simulink model "UrbanPHIL"  (Simulink 8.1)
settings: Solver=ode1  StartTime=0.0  StopTime=inf  FixedStep=Ts  MaxStep=1e-3  RelTol=1e-3
PostLoadFcn:
  | NREL_Mode=1; BANSHEE_init;
InitFcn:
  | NREL_Mode=1; BANSHEE_init;
values from neighbouring files (symbols this model uses):
  Ts = 100E-6    (= 0.0001)    [BANSHEE_init.m]    (also in Ghost_init.m)
undefined symbols (not defined in the file or in its folder): Hydride, Left, Metal, Nickel, type, V
libraries: powerlib x50, rteventslib x26, rtio_opalrt_op5142ex1 x25, artemis x13, simulink x6, cables_lib x4, relay_housing_lib x3, rtlab x2, utility_service_lib x1, Feeder1_lib x1, Feeder2_lib x1, Feeder3_lib x1
(part 1 of 3)
settings Model: ARTEMISmethode_block_infos=$$__separator__$$UrbanPHIL/ARTEMIS Guide$$__separator__$$  Creator=RE25624  LastModifiedBy=pkoralew  BufferReuse=off
settings SolverCC: ZeroCrossAlgorithm=Adaptive
settings DataIOCC: ExternalInput=getinputstruct(op_snapshot1)  InitialState=getstatestruct(op_snapshot1)  LimitDataPoints=off  MaxDataPoints=90060  SignalLoggingSaveFormat=Dataset  SaveOutput=off  SignalLogging=off  DSMLogging=off  SaveTime=off  OutputSaveName=result
settings OptimizationCC: BlockReduction=off  OptimizeBlockIOStorage=off  BufferReuse=off  ExpressionFolding=off  LocalBlockOutputs=off
settings DebuggingCC: MaxConsecutiveZCsMsg=warning  IgnoredZcDiagnostic=none  SolverPrmCheckMsg=none  MultiTaskRateTransMsg=warning  FcnCallInpInsideContextMsg=EnableAllAsWarning  FrameProcessingCompatibilityMsg=error  ModelReferenceExtraNoncontSigs=warning  StrictBusMsg=None
settings ModelReferenceCC: UpdateModelReferenceTargets=IfOutOfDate
settings SFSimCC: SFSimEcho=off
settings GRTTargetCC: CodeReplacementLibrary=C89/C90 (ANSI)

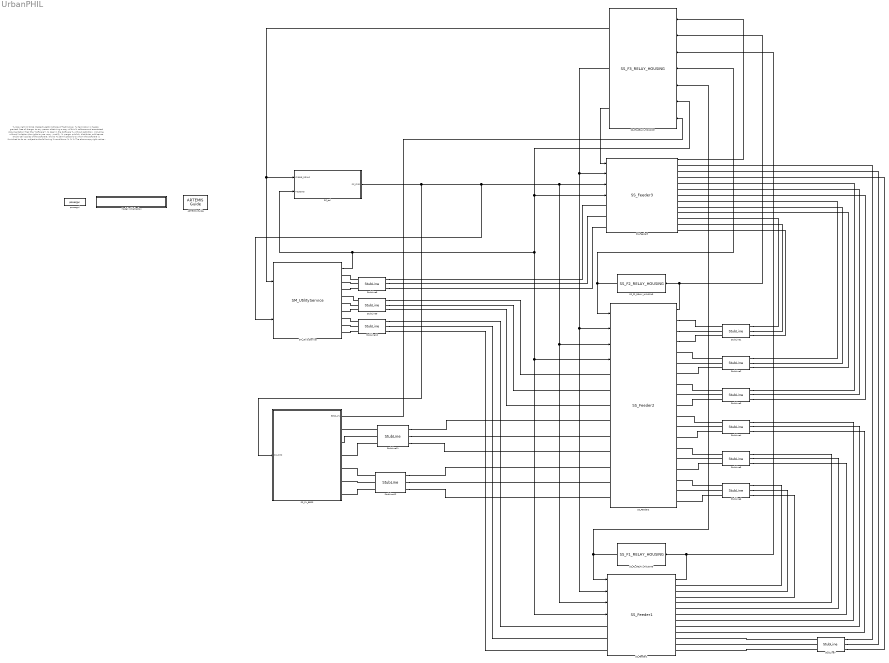
== system UrbanPHIL ==
  note: % Copyright (c) 2016 Massachusetts Institute of Technology
      | % Permission is hereby granted, free of charge, to any person obtaining a copy of this
      | % software and associated documentation files (the "Software"), to deal in the Software
      | % without restriction, including without limitation the rights to use, copy, modify,
      | % merge, publish, distribute, sublicense, and/or sell copies of the Software, and to
      | % permit persons to whom the Software is furnished to do so, subject to the following
      | % conditions:
      | %
      | %
      | % The above copyright notice and this permission notice shall be included in
      | % all copies or substantial portions of the Software.
      | %
      | % THE SOFTWARE IS PROVIDED "AS IS", WITHOUT WARRANTY OF ANY KIND, EXPRESS OR IMPLIED,
      | % INCLUDING BUT NOT LIMITED TO THE WARRANTIES OF MERCHANTABILITY, FITNESS FOR A
      | % PARTICULAR PURPOSE AND NONINFRINGEMENT. IN NO EVENT SHALL THE AUTHORS OR COPYRIGHT
      | % HOLDERS BE LIABLE FOR ANY CLAIM, DAMAGES OR OTHER LIABILITY, WHETHER IN AN ACTION
      | % OF CONTRACT, TORT OR OTHERWISE, ARISING FROM, OUT OF OR IN CONNECTION WITH THE
      | % SOFTWARE OR THE USE OR OTHER DEALINGS IN THE SOFTWARE.
      | %
      | %
      | %%
  ARTEMIS Guide : artemis/ARTEMIS/ARTEMIS Guide  Tag=FTSSmethode_opal_4hx0r99  Description=5.0_z1  lock=on  Ts=Ts  opt=art5  dyna=off  nb_perm=4  RT_fullcomp=off  ssn=on  ssn_itvc=off  ssn_ivic=off  ssn_ext=off  ssn_solver=Art5 with Backward Euler nodal interface  ssn_impulse=off  ssn_quasimpulse=off  ssn_impulse_loop=5  paraExtinctionThy=off  Thy_Impulse=on  dtc=Off  dtc_opt=normal  ao=on  simtype=off  ct_mac=off  lin_mov=off  lsp=[0.001 2]  spike_skip=Disabled  dtc_extra=1  dtc_sws=normal  dtc_pied=0.5  SPSRulesBlock=SPSRules  tre=on  ctmm=off  LF=off  dpl_type=ARTEMiS DPL  rlc_type=off  custom_type=off  para=on  ssn_ImpulseLoopBlockedStateUpdate=5  ssn_mov_iter_number=5  ssn_switch_iter_number=5
  Model Initialization : Subsystem  AncestorBlock=artemis/Tools /Misc/Model Initialization  mask(Model Functions){InitFcnX=NREL_Mode=1; BANSHEE_init;, prel=off, posl=on, inif=on, strf=off}
      mask prompts: InitFcnX "Initialisation"; prel "Preload Function"; posl "PostLoad Function"; inif "InitFcn"; strf "StartFcn"
      mask init:
      | currentBlock = gcb;
      | root = bdroot(currentBlock);
      | 
      | if ~strcmp(get_param(root,'BlockDiagramType'),'library')
      |     if prel==1
      |         set_param(root, 'PreLoadFcn', InitFcnX);
      |     else
      |         set_param(root, 'PreLoadFcn', '');
      |     end
      |     if inif==1
      |         set_param(root, 'InitFcn', InitFcnX);
      |     else
      |         set_param(root, 'InitFcn', '');
      |     end
      |     if strf==1
      |         set_param(root, 'StartFcn', InitFcnX);
      |     else
      |         set_param(root, 'StartFcn', '');
      |     end
      |     if posl==1
      |         set_param(root, 'PostLoadFcn', InitFcnX);
      |     else
      |         set_param(root, 'PostLoadFcn', '');
      |     end
      | end
      | 
      | pos = get_param(currentBlock, 'Position');
      | width = pos(3) - pos(1); height = pos(4) - pos(2);
      | txt = [ upper(root) '\n' '- InitFcn. . . . . '  get_param(root, 'InitFcn') ];
      settings: CopyFcn=set_param(gcb,'LinkStatus','inactive')
      mask Display: text(5, height*0.5, txt, 'horizontalAlignment', 'left', 'verticalAlignment', 'middle') ;
  SC_ctrl : Subsystem
  SM_UtilityService : utility_service_lib/SM_UtilityService
  SS_F1_RELAY_HOUSING : relay_housing_lib/SS_F1_RELAY_HOUSING
  SS_F2_RELAY_HOUSING : relay_housing_lib/SS_F2_RELAY_HOUSING
  SS_F3_RELAY_HOUSING : relay_housing_lib/SS_F3_RELAY_HOUSING
  SS_Feeder1 : Feeder1_lib/SS_Feeder1
  SS_Feeder2 : Feeder2_lib/SS_Feeder2
  SS_Feeder3 : Feeder3_lib/SS_Feeder3
  SS_PV_BESS : Subsystem
  StubLine1 : artemis/ARTEMIS/StubLine  Phases=3  pu=off  L=1500 * 9.43453e-08 / 2  Lpu=0.08  R=1500 * 2.28409e-5 / 2  Rpu=0.002  S_base=450e6/3  V_base=230e3/sqrt(3)  F_base=60  Ts=Ts
  StubLine10 : artemis/ARTEMIS/StubLine  Phases=3  pu=on  L=1500 * 9.43453e-08 / 2  Lpu=0.08  R=1500 * 2.28409e-5 / 2  Rpu=0.002  S_base=50e6/3  V_base=13.8e3/sqrt(3)  F_base=60  Ts=Ts
  StubLine11 : artemis/ARTEMIS/StubLine  Phases=3  pu=off  L=100 * 9.43453e-08  Lpu=0.08  R=100 * 2.28409e-5  Rpu=0.002  S_base=450e6/3  V_base=230e3/sqrt(3)  F_base=60  Ts=Ts
  StubLine12 : artemis/ARTEMIS/StubLine  Phases=3  pu=off  L=100 * 9.43453e-08  Lpu=0.08  R=100 * 2.28409e-5  Rpu=0.002  S_base=450e6/3  V_base=230e3/sqrt(3)  F_base=60  Ts=Ts
  StubLine2 : artemis/ARTEMIS/StubLine  Phases=3  pu=off  L=1500 * 9.43453e-08 / 2  Lpu=0.08  R=1500 * 2.28409e-5 / 2  Rpu=0.002  S_base=450e6/3  V_base=230e3/sqrt(3)  F_base=60  Ts=Ts
  StubLine3 : artemis/ARTEMIS/StubLine  Phases=3  pu=off  L=1500 * 9.43453e-08 / 2  Lpu=0.08  R=1500 * 2.28409e-5 / 2  Rpu=0.002  S_base=450e6/3  V_base=230e3/sqrt(3)  F_base=60  Ts=Ts
  StubLine4 : artemis/ARTEMIS/StubLine  Phases=3  pu=off  L=1000 * 9.43453e-08 / 2  Lpu=0.08  R=1000 * 2.28409e-5 / 2  Rpu=0.002  S_base=450e6/3  V_base=230e3/sqrt(3)  F_base=60  Ts=Ts
  StubLine5 : artemis/ARTEMIS/StubLine  Phases=3  pu=off  L=2000 * 9.43453e-08 / 2  Lpu=0.08  R=2000 * 2.28409e-5 / 2  Rpu=0.002  S_base=450e6/3  V_base=230e3/sqrt(3)  F_base=60  Ts=Ts
  StubLine6 : artemis/ARTEMIS/StubLine  Phases=3  pu=off  L=2000 * 9.43453e-08 / 2  Lpu=0.08  R=2000 * 2.28409e-5 / 2  Rpu=0.002  S_base=450e6/3  V_base=230e3/sqrt(3)  F_base=60  Ts=Ts
  StubLine7 : artemis/ARTEMIS/StubLine  Phases=3  pu=off  L=2000 * 9.43453e-08 / 2  Lpu=0.08  R=2000 * 2.28409e-5 / 2  Rpu=0.002  S_base=450e6/3  V_base=230e3/sqrt(3)  F_base=60  Ts=Ts
  StubLine8 : artemis/ARTEMIS/StubLine  Phases=3  pu=on  L=1500 * 9.43453e-08 / 2  Lpu=0.08  R=1500 * 2.28409e-5 / 2  Rpu=0.002  S_base=50e6/3  V_base=13.8e3/sqrt(3)  F_base=60  Ts=Ts
  StubLine9 : artemis/ARTEMIS/StubLine  Phases=3  pu=on  L=1500 * 9.43453e-08 / 2  Lpu=0.08  R=1500 * 2.28409e-5 / 2  Rpu=0.002  S_base=50e6/3  V_base=13.8e3/sqrt(3)  F_base=60  Ts=Ts
  powergui : powerlib/powergui  Priority=2  SimulationMode=Discrete  SolverType=Tustin  SampleTime=Ts  frequency=60  SPID=off  DisableSnubberDevices=off  DisableRonSwitches=off  DisableVfSwitches=off  SwTol=0  Interpol=off  DisplayEquations=off  frequencyindice=0  Pbase=100e6  ErrMax=1e-4  Iterations=50  UnitsV=kV  UnitsW=MW  FunctionMessages=off  echomessages=off  HookPort=off  EnableUseOfTLC=off  x0status=blocks  RestoreLinks=warning  ResistiveCurrentMeasurement=off  Frange=logspace(0,3,50)  Ylog=off  Xlog=off  ShowGrid=off  save=off  variable=ZData  structure=0  ZoomFFT=on  StartTime=0.0  cycles=2  DisplayStyle=off  fundamental=60  FreqAxis=off  MaxFrequency=1000  frequencyindicesteady=1  RmsSteady=1  display=off  Ts=0  methode=off
  wires:
  SS_Feeder3/1 -> SS_F3_RELAY_HOUSING/1
  SS_F3_RELAY_HOUSING/3 -> SS_Feeder3/1
  SS_F1_RELAY_HOUSING/1 -> SS_F3_RELAY_HOUSING/5, SS_Feeder1/1
  SS_F2_RELAY_HOUSING/1 -> SS_F3_RELAY_HOUSING/4, SS_Feeder2/1
  SS_Feeder1/1 -> SS_F3_RELAY_HOUSING/3, SS_F1_RELAY_HOUSING/1
  SS_Feeder2/1 -> SS_F3_RELAY_HOUSING/2, SS_F2_RELAY_HOUSING/1
  SS_F3_RELAY_HOUSING/2 -> SS_Feeder1/2, SS_Feeder2/2, SS_Feeder3/2
  SM_UtilityService/1 -> SC_ctrl/2(TestData), SS_Feeder1/4, SS_Feeder2/4, SS_F3_RELAY_HOUSING/6, SS_Feeder3/4
  SS_F3_RELAY_HOUSING/1 -> SC_ctrl/1(CMBNE_SGNLS), SM_UtilityService/1
  SC_ctrl/1(SC_CMD) -> SS_PV_BESS/1(SC_CMD), SM_UtilityService/2, SS_Feeder1/3, SS_Feeder2/3, SS_Feeder3/3
  SS_PV_BESS/1(BESS_PV) -> SS_F3_RELAY_HOUSING/7
  connections:
  SS_Feeder2/RConn2 -- StubLine1/LConn2
  SS_Feeder2/RConn1 -- StubLine1/LConn1
  SS_Feeder2/RConn3 -- StubLine1/LConn3
  StubLine2/LConn2 -- SS_Feeder2/RConn5
  StubLine2/LConn3 -- SS_Feeder2/RConn6
  StubLine2/LConn1 -- SS_Feeder2/RConn4
  StubLine3/LConn2 -- SS_Feeder2/RConn8
  StubLine3/LConn1 -- SS_Feeder2/RConn7
  StubLine3/LConn3 -- SS_Feeder2/RConn9
  StubLine4/LConn3 -- SS_Feeder2/RConn12
  StubLine4/LConn2 -- SS_Feeder2/RConn11
  StubLine4/LConn1 -- SS_Feeder2/RConn10
  StubLine7/LConn3 -- SS_Feeder1/RConn12
  StubLine7/LConn2 -- SS_Feeder1/RConn11
  StubLine7/LConn1 -- SS_Feeder1/RConn10
  StubLine5/LConn2 -- SS_Feeder2/RConn14
  StubLine5/LConn1 -- SS_Feeder2/RConn13
  StubLine5/LConn3 -- SS_Feeder2/RConn15
  StubLine6/LConn3 -- SS_Feeder2/RConn18
  StubLine6/LConn2 -- SS_Feeder2/RConn17
  StubLine6/LConn1 -- SS_Feeder2/RConn16
  StubLine6/RConn1 -- SS_Feeder1/RConn1
  StubLine6/RConn2 -- SS_Feeder1/RConn2
  StubLine6/RConn3 -- SS_Feeder1/RConn3
  StubLine5/RConn1 -- SS_Feeder1/RConn4
  StubLine5/RConn2 -- SS_Feeder1/RConn5
  StubLine5/RConn3 -- SS_Feeder1/RConn6
  StubLine4/RConn1 -- SS_Feeder1/RConn7
  StubLine4/RConn2 -- SS_Feeder1/RConn8
  StubLine4/RConn3 -- SS_Feeder1/RConn9
  StubLine3/RConn3 -- SS_Feeder3/RConn6
  StubLine3/RConn2 -- SS_Feeder3/RConn5
  StubLine3/RConn1 -- SS_Feeder3/RConn4
  StubLine2/RConn3 -- SS_Feeder3/RConn9
  StubLine2/RConn2 -- SS_Feeder3/RConn8
  StubLine2/RConn1 -- SS_Feeder3/RConn7
  StubLine1/RConn3 -- SS_Feeder3/RConn12
  StubLine1/RConn2 -- SS_Feeder3/RConn11
  StubLine1/RConn1 -- SS_Feeder3/RConn10
  StubLine7/RConn1 -- SS_Feeder3/RConn1
  StubLine7/RConn2 -- SS_Feeder3/RConn2
  StubLine7/RConn3 -- SS_Feeder3/RConn3
  StubLine8/LConn1 -- SM_UtilityService/RConn1
  StubLine8/LConn2 -- SM_UtilityService/RConn2
  StubLine8/LConn3 -- SM_UtilityService/RConn3
  StubLine9/LConn2 -- SM_UtilityService/RConn5
  StubLine9/LConn3 -- SM_UtilityService/RConn6
  StubLine9/LConn1 -- SM_UtilityService/RConn4
  StubLine10/LConn2 -- SM_UtilityService/RConn8
  StubLine10/LConn3 -- SM_UtilityService/RConn9
  StubLine10/LConn1 -- SM_UtilityService/RConn7
  StubLine8/RConn3 -- SS_Feeder3/LConn3
  StubLine8/RConn2 -- SS_Feeder3/LConn2
  StubLine8/RConn1 -- SS_Feeder3/LConn1
  StubLine10/RConn1 -- SS_Feeder1/LConn1
  StubLine10/RConn2 -- SS_Feeder1/LConn2
  StubLine10/RConn3 -- SS_Feeder1/LConn3
  StubLine9/RConn1 -- SS_Feeder2/LConn1
  StubLine9/RConn2 -- SS_Feeder2/LConn2
  StubLine9/RConn3 -- SS_Feeder2/LConn3
  StubLine11/LConn2 -- SS_PV_BESS/RConn2
  StubLine11/LConn1 -- SS_PV_BESS/RConn1
  StubLine11/LConn3 -- SS_PV_BESS/RConn3
  StubLine11/RConn2 -- SS_Feeder2/LConn5
  StubLine11/RConn3 -- SS_Feeder2/LConn6
  StubLine11/RConn1 -- SS_Feeder2/LConn4
  StubLine12/LConn2 -- SS_PV_BESS/RConn5
  StubLine12/LConn1 -- SS_PV_BESS/RConn4
  StubLine12/LConn3 -- SS_PV_BESS/RConn6
  StubLine12/RConn2 -- SS_Feeder2/LConn8
  StubLine12/RConn1 -- SS_Feeder2/LConn7
  StubLine12/RConn3 -- SS_Feeder2/LConn9

== system UrbanPHIL/Model Initialization ==

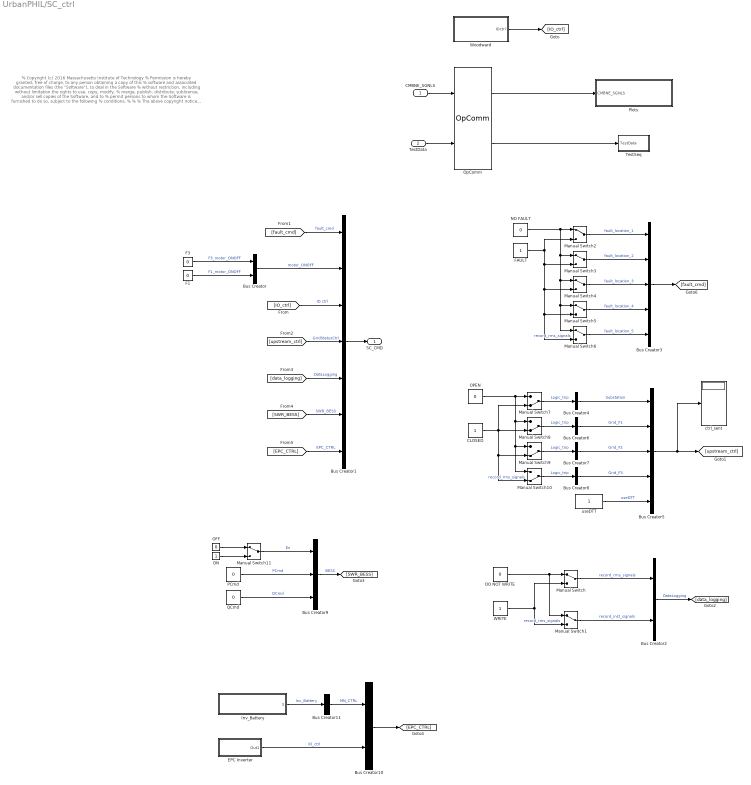
== system UrbanPHIL/SC_ctrl ==
  note: % Copyright (c) 2016 Massachusetts Institute of Technology
      | % Permission is hereby granted, free of charge, to any person obtaining a copy of this
      | % software and associated documentation files (the "Software"), to deal in the Software
      | % without restriction, including without limitation the rights to use, copy, modify,
      | % merge, publish, distribute, sublicense, and/or sell copies of the Software, and to
      | % permit persons to whom the Software is furnished to do so, subject to the following
      | % conditions:
      | %
      | %
      | % The above copyright notice and this permission notice shall be included in
      | % all copies or substantial portions of the Software.
      | %
      | % THE SOFTWARE IS PROVIDED "AS IS", WITHOUT WARRANTY OF ANY KIND, EXPRESS OR IMPLIED,
      | % INCLUDING BUT NOT LIMITED TO THE WARRANTIES OF MERCHANTABILITY, FITNESS FOR A
      | % PARTICULAR PURPOSE AND NONINFRINGEMENT. IN NO EVENT SHALL THE AUTHORS OR COPYRIGHT
      | % HOLDERS BE LIABLE FOR ANY CLAIM, DAMAGES OR OTHER LIABILITY, WHETHER IN AN ACTION
      | % OF CONTRACT, TORT OR OTHERWISE, ARISING FROM, OUT OF OR IN CONNECTION WITH THE
      | % SOFTWARE OR THE USE OR OTHER DEALINGS IN THE SOFTWARE.
      | %
      | %
      | %%
  CMBNE_SGNLS : Inport
  TestData : Inport  Port=2
  Bus Creator : BusCreator  Inputs=2
  Bus Creator1 : BusCreator  Inputs=7
  Bus Creator10 : BusCreator  Inputs=2
  Bus Creator{4,6..8,11} (5 alike) : BusCreator  Inputs=1
  Bus Creator2 : BusCreator  Inputs=2
  Bus Creator3 : BusCreator  Inputs=5
  Bus Creator5 : BusCreator  Inputs=5
  Bus Creator9 : BusCreator  Inputs=3
  CLOSED : Constant
  DO NOT WRITE : Constant  Value=0
  EPC Inverter : Subsystem
  F1 : Constant  Value=0
  F3 : Constant  Value=0
  FAULT : Constant
  Inv_Battery : Subsystem
  Manual Switch{,1..6,11} (8 alike) : ManualSwitch
  Manual Switch{7..10} (4 alike) : ManualSwitch  CurrentSetting=0
  NO FAULT : Constant  Value=0
  OFF : Constant  Value=0
  ON : Constant
  OPEN : Constant  Value=0
  OpComm : rtlab/OpComm  nbport=2  groupe_acq=1  subsys_rate=0  st=0  Synchronization=on  Interpolation=on  Threshold=1.0  Missed_Data=off  Sim_Time=off  Samples=off  dynSigOut=off  from_console=0  warning_done=off  writeOpCommFile=off  Offset=off
  PCmd : Constant  Value=0  SampleTime=Ts
  Plots : Subsystem
  QCmd : Constant  Value=0  SampleTime=Ts
  TestSeq : Subsystem
  WRITE : Constant
  Woodward : Subsystem
  ctrl_sent : Display
  useDTT : Constant
  SC_CMD : Outport
  wires:
  CMBNE_SGNLS/1 -> OpComm/1
  Bus Creator1/1 -> SC_CMD/1
  [IO_ctrl] -> Bus Creator1/3  "IO ctrl"
  Woodward/1(IOctrl) -> [IO_ctrl]
  [fault_cmd] -> Bus Creator1/1  "fault_cmd"
  Bus Creator/1 -> Bus Creator1/2  "motor_ONOFF"
  F3/1 -> Bus Creator/1  "F3_motor_ONOFF"
  F1/1 -> Bus Creator/2  "F1_motor_ONOFF"
  [upstream_ctrl] -> Bus Creator1/4  "GridStatusCtrl"
  Manual Switch/1 -> Bus Creator2/1  "record_rms_signals"
  Manual Switch1/1 -> Bus Creator2/2  "record_inst_signals"
  Bus Creator2/1 -> [data_logging]  "DataLogging"
  OpComm/1 -> Plots/1(CMBNE_SGNLS)
  OpComm/2 -> TestSeq/1(TestData)
  TestData/1 -> OpComm/2
  WRITE/1 -> Manual Switch1/2, Manual Switch/2  "record_rms_signals"
  DO NOT WRITE/1 -> Manual Switch1/1, Manual Switch/1
  Bus Creator3/1 -> [fault_cmd]
  Manual Switch2/1 -> Bus Creator3/1  "fault_location_1"
  Manual Switch6/1 -> Bus Creator3/5  "fault_location_5"
  Manual Switch3/1 -> Bus Creator3/2  "fault_location_2"
  Manual Switch4/1 -> Bus Creator3/3  "fault_location_3"
  Manual Switch5/1 -> Bus Creator3/4  "fault_location_4"
  NO FAULT/1 -> Manual Switch6/1, Manual Switch5/1, Manual Switch4/1, Manual Switch3/1, Manual Switch2/1
  FAULT/1 -> Manual Switch2/2, Manual Switch6/2, Manual Switch5/2, Manual Switch4/2, Manual Switch3/2  "record_rms_signals"
  Manual Switch10/1 -> Bus Creator8/1  "Logic_trip"
  Manual Switch9/1 -> Bus Creator7/1  "Logic_trip"
  Bus Creator5/1 -> ctrl_sent/1, [upstream_ctrl]
  Manual Switch8/1 -> Bus Creator6/1  "Logic_trip"
  Bus Creator4/1 -> Bus Creator5/1  "Substation"
  Manual Switch7/1 -> Bus Creator4/1  "Logic_trip"
  Bus Creator8/1 -> Bus Creator5/4  "Grid_F3"
  Bus Creator7/1 -> Bus Creator5/3  "Grid_F2"
  Bus Creator6/1 -> Bus Creator5/2  "Grid_F1"
  useDTT/1 -> Bus Creator5/5  "useDTT"
  OPEN/1 -> Manual Switch7/1, Manual Switch8/1, Manual Switch9/1, Manual Switch10/1
  CLOSED/1 -> Manual Switch7/2, Manual Switch8/2, Manual Switch9/2, Manual Switch10/2  "record_rms_signals"
  Manual Switch11/1 -> Bus Creator9/1  "En"
  PCmd/1 -> Bus Creator9/2  "PCmd"
  QCmd/1 -> Bus Creator9/3  "QCmd"
  ON/1 -> Manual Switch11/2
  OFF/1 -> Manual Switch11/1
  [data_logging] -> Bus Creator1/5  "DataLogging"
  Bus Creator9/1 -> [SWR_BESS]  "BESS"
  [SWR_BESS] -> Bus Creator1/6  "SWR_BESS"
  EPC Inverter/1(Out1) -> Bus Creator10/2  "IO_ctrl"
  Inv_Battery/1(S) -> Bus Creator11/1  "Inv_Battery"
  Bus Creator11/1 -> Bus Creator10/1  "MN_CTRL"
  Bus Creator10/1 -> [EPC_CTRL]
  [EPC_CTRL] -> Bus Creator1/7  "EPC_CTRL"

== system UrbanPHIL/SS_PV_BESS ==
  SC_CMD : Inport
  BESS : BESS_lib/BESS
  Bus Creator6 : BusCreator  Inputs=2
  Bus Selector7 : BusSelector  OutputSignals=SWR_BESS,EPC_CTRL
  C1 : cables_lib/500kcmil-Mutual  length=10  par_sets=1  ratio=3
  C202 : cables_lib/500kcmil-Mutual  length=10  par_sets=1  ratio=3
  EPC : Subsystem
  Memory : Memory
  OpComm3 : rtlab/OpComm  nbport=1  groupe_acq=1  subsys_rate=0  st=0  Synchronization=on  Interpolation=on  Threshold=1.0  Missed_Data=off  Sim_Time=off  Samples=off  dynSigOut=off  from_console=1  warning_done=off  writeOpCommFile=off  Offset=off
  A_PV : PMIOPort  Port=1  Side=Right
  B_PV : PMIOPort  Port=2  Side=Right
  C_PV : PMIOPort  Port=3  Side=Right
  A_BESS : PMIOPort  Port=4  Side=Right
  B_BESS : PMIOPort  Port=5  Side=Right
  C_BESS : PMIOPort  Port=6  Side=Right
  BESS_PV : Outport
  wires:
  SC_CMD/1 -> OpComm3/1
  OpComm3/1 -> Bus Selector7/1
  Bus Selector7/1 -> [SWR_BESS]  "<SWR_BESS>"
  [SWR_BESS] -> BESS/1
  BESS/1 -> [BESS_MS]
  Memory/1 -> BESS_PV/1
  Bus Creator6/1 -> Memory/1
  [BESS_MS] -> Bus Creator6/1  "BESS"
  EPC/1(monitoring) -> [EPC_MS]
  [EPC_MS] -> Bus Creator6/2  "EPC"
  [EPC_CTRL] -> EPC/1(FROM_SC)
  Bus Selector7/2 -> [EPC_CTRL]  "<EPC_CTRL>"
  connections:
  B_BESS/RConn1 -- C1/RConn2
  C_BESS/RConn1 -- C1/RConn3
  A_BESS/RConn1 -- C1/RConn1
  B_PV/RConn1 -- C202/RConn2
  C_PV/RConn1 -- C202/RConn3
  A_PV/RConn1 -- C202/RConn1
  BESS/RConn2 -- C202/LConn2
  BESS/RConn3 -- C202/LConn3
  BESS/RConn1 -- C202/LConn1
  EPC/LConn1 -- C1/LConn1
  EPC/LConn2 -- C1/LConn2
  EPC/LConn3 -- C1/LConn3

== system UrbanPHIL/SC_ctrl/EPC Inverter ==
  note: This corresponds to
      | the DIO Enable MCB
  note: Op_Mode:
      | 0 = Relay Functions
      | 1 = Close Breaker
      | 2 = Open Breaker
  16Din/16Dout GR3 : Subsystem
  16PWMIn/16PWMout GR3 : Subsystem
  16TSDIn/16 TSDOut GR3 : Subsystem
  Brk1 Grid : Constant  Value=2
  Brk10 Gen 1 Busbar : Constant
  Brk2 Load 1 : Constant  Value=0
  Brk3 Inv MX1 : Constant  Value=2
  Brk4 Gen 1 MCB : Constant  Value=2
  Brk5 Gen 2 LCB : Constant  Value=0
  Brk6 Gen 1 LCB : Constant  Value=0
  Brk7 Gen 2 GCB : Constant
  Brk8 Gen 1 GCB : Constant
  Brk9 Gen 2 Busbar : Constant
  Bus Creator1 : BusCreator  Inputs=3
  Bus Creator2 : BusCreator  Inputs=2
  Bus Creator3 : BusCreator  Inputs=14
  Wood MCB Enable : Constant  Value=0
  bias_ctrl : Constant
  control_mode : Constant
  gen_enable : Constant
  Out1 : Outport
  wires:
  Brk10 Gen 1 Busbar/1 -> Bus Creator3/10  "Gen1_Busbar"
  Brk9 Gen 2 Busbar/1 -> Bus Creator3/9  "Gen2_Busbar"
  Brk8 Gen 1 GCB/1 -> Bus Creator3/8  "Gen1_GCB"
  Brk7 Gen 2 GCB/1 -> Bus Creator3/7  "Gen2_GCB"
  Brk6 Gen 1 LCB/1 -> Bus Creator3/6  "Load 3"
  Brk5 Gen 2 LCB/1 -> Bus Creator3/5  "Load 2"
  Wood MCB Enable/1 -> Bus Creator3/14  "Wood_MCB_enable"
  Bus Creator2/1 -> Out1/1
  bias_ctrl/1 -> Bus Creator3/13  "Gen_bias_enable"
  gen_enable/1 -> Bus Creator3/12  "Gen2_enable"
  control_mode/1 -> Bus Creator3/11  "Wood_DIO"
  Brk4 Gen 1 MCB/1 -> Bus Creator3/4  "Gen1_MCB"
  Brk3 Inv MX1/1 -> Bus Creator3/3  "MX1"
  Brk2 Load 1/1 -> Bus Creator3/2  "Load 1"
  Brk1 Grid/1 -> Bus Creator3/1  "Grid"
  Bus Creator3/1 -> Bus Creator2/2  "test_controls"
  Bus Creator1/1 -> Bus Creator2/1  "DOUT GR3"
  16PWMIn/16PWMout GR3/1(To PWMOut) -> Bus Creator1/3  "16 PWMOUT GR3"
  16TSDIn/16 TSDOut GR3/1(TSDout) -> Bus Creator1/2  "16 TSDOUT GR3"
  16Din/16Dout GR3/1(Dout) -> Bus Creator1/1  "16 DOUT GR3"

== system UrbanPHIL/SC_ctrl/Inv_Battery ==
  note: Make this 1 to allow
      | the external signals.
  note: Remote Sense =>1
      | Use Remote Sense EPyQ
      | Sync or not => grid forming/grid following
  note: 0=> Local
      | 1=> Remote
  note: 0=> No Console
      | 1=> Console Ctrl
  note: 1 => Sig 1 is Bot then Sig 2 is Top
      | 0 => Sig 1 is Top then Sig 2 is Bot
  note: 0=> RTE
      | 1=> Simulink
  note: LSB
  note: MSB
  note: 1111: RTE TSD Signal Modulation External
      | 0111: RTE Signal Modulation Internal
      | X011: Sin Tri Modulatiion Internal
      | XX01: Digital Inputs
      | XXX0; Open Switches
  note: MCB
  note: GCB
  note: 1 => Closed
      | 2=> Open
  note: ~ 2.5 sec to get
      | to rated voltage
  note: RTE Internal
      | All 0 and one 1
  note: Internal = 0
      | External = 1
  Bus Creator : BusCreator  Inputs=8
  Bus Creator1 : BusCreator  Inputs=5
  Console : Constant  Value=0
  DC Contactor : Constant  Value=0
  Enable PWM{0..3} (4 alike) : Constant
  MX1 : Constant  Value=2
  MX2 : Constant  Value=2
  Precharge : Constant  Value=0
  Sense : Constant  Value=0
  Signal Mapping : Constant
  Simulink : Constant  Value=0
  S : Outport
  wires:
  Sense/1 -> Bus Creator/8  "LOCALvsREMOTE"
  Console/1 -> Bus Creator/7  "Console_Ctrl"
  Signal Mapping/1 -> Bus Creator1/5  "Ext_PWM_RTE_Signal"
  Simulink/1 -> Bus Creator/6  "RTEvsSPS"
  Enable PWM3/1 -> Bus Creator1/1
  Enable PWM2/1 -> Bus Creator1/2
  Enable PWM1/1 -> Bus Creator1/3
  Enable PWM0/1 -> Bus Creator1/4
  Bus Creator1/1 -> Bus Creator/1  "Enable PWM"
  MX2/1 -> Bus Creator/5  "MX2"
  MX1/1 -> Bus Creator/4  "MX1"
  DC Contactor/1 -> Bus Creator/3  "DC_Contactor"
  Precharge/1 -> Bus Creator/2  "Precharge"
  Bus Creator/1 -> S/1

== system UrbanPHIL/SC_ctrl/Plots ==
  note: VRMSLL
      | Hz
      | kW
      | kVAR
  CMBNE_SGNLS : Inport
  Bus Selector1 : BusSelector  OutputSignals=F1_MS_IN.DIESEL_DATA.DIESEL_GCB.VRMSLL,F1_MS_IN.DIESEL_DATA.DIESEL_GCB.Freq,F1_MS_IN.DIESEL_DATA.DIESEL_GCB.kw,F1_MS_IN.DIESEL_DATA.DIESEL_GCB.kvar  OutputAsBus=on
  Bus Selector2 : BusSelector  OutputSignals=F3_MS_IN.NG_CHP_DATA.NG_CHP_GCB.VRMSLL,F3_MS_IN.NG_CHP_DATA.NG_CHP_GCB.Freq,F3_MS_IN.NG_CHP_DATA.NG_CHP_GCB.kw,F3_MS_IN.NG_CHP_DATA.NG_CHP_GCB.kvar  OutputAsBus=on
  Bus Selector3 : BusSelector  OutputSignals=PCC_DATA_OUT.F3_PCC.VRMSLL,PCC_DATA_OUT.F3_PCC.Freq,PCC_DATA_OUT.F3_PCC.kw,PCC_DATA_OUT.F3_PCC.kvar  OutputAsBus=on
  Bus Selector4 : BusSelector  OutputSignals=PCC_DATA_OUT.F2_PCC.VRMSLL,PCC_DATA_OUT.F2_PCC.Freq,PCC_DATA_OUT.F2_PCC.kw,PCC_DATA_OUT.F2_PCC.kvar  OutputAsBus=on
  Bus Selector5 : BusSelector  OutputSignals=PCC_DATA_OUT.F1_PCC.VRMSLL,PCC_DATA_OUT.F1_PCC.Freq,PCC_DATA_OUT.F1_PCC.kw,PCC_DATA_OUT.F1_PCC.kvar  OutputAsBus=on
  Bus Selector6 : BusSelector  OutputSignals=BESS_PV.BESS.kw,BESS_PV.BESS.kvar,BESS_PV.BESS.Freq  OutputAsBus=on
  Bus Selector7 : BusSelector  OutputSignals=BESS_PV.EPC.BESS_MX1.VRMSLL,BESS_PV.EPC.BESS_MX1.Freq,BESS_PV.EPC.BESS_MX1.kw,BESS_PV.EPC.BESS_MX1.kvar  OutputAsBus=on
  Bus Selector8 : BusSelector  OutputSignals=BESS_PV.EPC.BESS_MX1.cb_ms.Iabc,BESS_PV.EPC.BESS_MX1.cb_ms.Vabc_line
  CHP : Display
  Diesel : Display
  EPC_BESS : Display
  EPC_BESS Scope : Scope  NumInputPorts=2
      settings: YMin=-5~-5  YMax=5~5
  F1 : Display
  F2 : Display
  F3 : Display
  SWR_BESS : Display
  wires:
  Bus Selector5/1 -> F1/1
  Bus Selector4/1 -> F2/1
  Bus Selector3/1 -> F3/1
  Bus Selector1/1 -> Diesel/1
  Bus Selector2/1 -> CHP/1
  CMBNE_SGNLS/1 -> [CMBNE_SGNLS]
  [CMBNE_SGNLS] -> Bus Selector5/1
  [CMBNE_SGNLS] -> Bus Selector4/1
  [CMBNE_SGNLS] -> Bus Selector3/1
  [CMBNE_SGNLS] -> Bus Selector2/1
  [CMBNE_SGNLS] -> Bus Selector1/1
  [CMBNE_SGNLS] -> Bus Selector6/1
  Bus Selector6/1 -> SWR_BESS/1
  [CMBNE_SGNLS] -> Bus Selector7/1
  Bus Selector7/1 -> EPC_BESS/1
  [CMBNE_SGNLS] -> Bus Selector8/1
  Bus Selector8/2 -> EPC_BESS Scope/2  "<Vabc_line>"
  Bus Selector8/1 -> EPC_BESS Scope/1  "<Iabc>"

== system UrbanPHIL/SC_ctrl/TestSeq ==
  TestData : Inport
  Bus Selector : BusSelector  OutputSignals=TestSeq.TimeStamp,TestSeq.fault_location_1,TestSeq.fault_location_2,TestSeq.fault_location_3,TestSeq.fault_location_4,TestSeq.fault_location_5,TestSeq.Cut_Grid_Power,TestSeq.Irradiance,TestSeq.motor_1,TestSeq.motor_2,TestSeq.Test3
  Display : Display
  Scope : Scope  NumInputPorts=10
      settings: YMin=-5~-5~-5~-5~-5~-5~-5~-5~-5~-5  YMax=5~5~5~5~5~5~5~5~5~5
  wires:
  TestData/1 -> Bus Selector/1
  Bus Selector/1 -> Display/1  "<TimeStamp>"
  Bus Selector/6 -> Scope/5  "<fault_location_5>"
  Bus Selector/5 -> Scope/4  "<fault_location_4>"
  Bus Selector/10 -> Scope/9  "<motor_2>"
  Bus Selector/2 -> Scope/1  "<fault_location_1>"
  Bus Selector/3 -> Scope/2  "<fault_location_2>"
  Bus Selector/8 -> Scope/7  "<Irradiance>"
  Bus Selector/9 -> Scope/8  "<motor_1>"
  Bus Selector/4 -> Scope/3  "<fault_location_3>"
  Bus Selector/7 -> Scope/6  "<Cut_Grid_Power>"
  Bus Selector/11 -> Scope/10  "<Test3>"

== system UrbanPHIL/SC_ctrl/Woodward ==
  16Din/16Dout GR3 : Subsystem
  Bus Creator2 : BusCreator  Inputs=1
  IOctrl : Outport
  wires:
  16Din/16Dout GR3/1(Dout) -> Bus Creator2/1  "16 DOUT GR3"
  Bus Creator2/1 -> IOctrl/1  "IO ctrl"

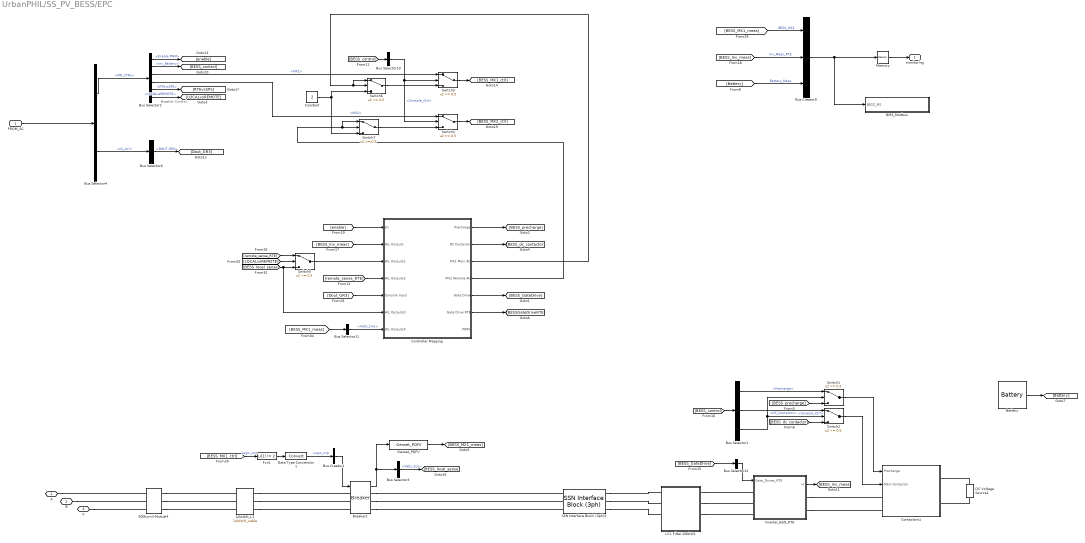
== system UrbanPHIL/SS_PV_BESS/EPC ==
  note: Breaker Control
  FROM_SC : Inport
  1/0AWG_L1 : cables_lib/1//0AWG_cable  length=1  par_sets=1
  500kcmil-Mutual4 : cables_lib/500kcmil-Mutual  length=50  par_sets=1  ratio=3
  BMS_Modbus : Subsystem
  Battery : electricdrivelib/Extra Sources/Battery  BatType=Nickel-Metal-Hydride  ShowDetailedParameters=off  NomV=1.2  NomQ=1.5  SOC=100  PresetModel=on  MaxQ=1.6154  FullV=1.4136  Dis_rate=0.3  R=0.008  Normal_OP=1.4423  expZone="[1.3017         0.3]"  Dis_Char=off  current=[1.5 3]  Units=Ampere-hour  Batt_Tr=30
  Breaker1 : breaker_lib/Breaker  Ts=Ts  mech_delay=0.0833
  Bus Creator1 : BusCreator  Inputs=1
  Bus Creator9 : BusCreator  Inputs=3
  Bus Selector1 : BusSelector  OutputSignals=Precharge,DC_Contactor,Console_Ctrl
  Bus Selector10 : BusSelector  OutputSignals=Console_Ctrl
  Bus Selector11 : BusSelector  OutputSignals=cb_ms.Vabc_line
  Bus Selector12 : BusSelector  OutputSignals=signal1,signal2,signal3,signal4,signal5,signal6  OutputAsBus=on
  Bus Selector2 : BusSelector  OutputSignals=Inv_Battery.Enable PWM,Inv_Battery,Inv_Battery.MX1,Inv_Battery.MX2,Inv_Battery.RTEvsSPS,Inv_Battery.LOCALvsREMOTE
  Bus Selector3 : BusSelector  OutputSignals=Vabc_bus
  Bus Selector4 : BusSelector  OutputSignals=MN_CTRL,IO_ctrl
  Bus Selector6 : BusSelector  OutputSignals=DOUT GR3
  Constant : Constant  Value=2
  Contactors1 : Subsystem
  Controller Mapping : Subsystem
  DC Voltage Source1 : powerlib/Electrical Sources/DC Voltage Source  Amplitude=800  Measurements=Voltage
  Data Type Conversion1 : DataTypeConversion
  Fcn1 : Fcn  Expr=u(1) != 2
  Genset_PQFV : PQFV_lib/Genset_PQFV  VRMSLL=480  Ts=Ts
  Inverter_Batt_RTE : Subsystem
  LCL Filter 200kW1 : Subsystem  mask(LCL Filter){filter_line_ind=50e-6, filter_line_res=0, filter_cap=650e-6, filter_cap_res=100e-3, filter_cap_bleed_res=75e3, filter_inv_ind=85e-6, filter_inv_res=0}
      mask prompts: filter_line_ind "Line Inductor (H)"; filter_line_res "Line Inductor Resistance (Ohm)"; filter_cap "Capacitor (F)"; filter_cap_res "Resistance with Capacitor (ohm)"; filter_cap_bleed_res "Resistance for Capacitor Discharge (ohm)"; filter_inv_ind "Inverter Inductor (H)"; filter_inv_res "Inverter Inductor Resistance (Ohm)"
      mask help: This filter is the LCL filter for the inverter.
  Memory : Memory
  SSN Interface Block (3ph)3 : ssn_lib/SSN Interface Block (3ph)  nb_phase=3  nb_port=2  p1_type=V-type(Left)  p2_type=V-type (Right)  p3_type=V-type(Left)  p4_type=V-type(Left)  p5_type=V-type(Left)  p6_type=V-type(Left)  p7_type=V-type(Left)  p8_type=V-type(Left)  p9_type=V-type(Left)  p10_type=V-type(Left)  p11_type=V-type(Left)  p12_type=V-type(Left)  p13_type=V-type(Left)  p14_type=V-type(Left)  p15_type=V-type(Left)  p16_type=V-type(Left)  I_port_shunt_resistance=1e9
  Switch{1..7} (7 alike) : Switch  Threshold=0.5
  A : PMIOPort  Port=1  Side=Left
  B : PMIOPort  Port=2  Side=Left
  C : PMIOPort  Port=3  Side=Left
  monitoring : Outport
  wires:
  Switch5/1 -> Controller Mapping/3(HIL Outputs1)
  Bus Selector12/1 -> Inverter_Batt_RTE/1(Gate_Drives_RTE)
  FROM_SC/1 -> Bus Selector4/1
  [BESS_MX1_ctrl] -> Fcn1/1  "Logic_trip"
  Fcn1/1 -> Data Type Conversion1/1
  Bus Selector3/1 -> [BESS_local_sense]  "<Vabc_bus>"
  Genset_PQFV/1 -> [BESS_MX1_meas]
  Breaker1/1 -> Genset_PQFV/1, Bus Selector3/1
  Data Type Conversion1/1 -> Bus Creator1/1  "Logic_trip"
  Bus Creator1/1 -> Breaker1/1
  [Battery] -> Bus Creator9/3  "Battery_Meas"
  [BESS_MX1_meas] -> Bus Creator9/1  "BESS_MX1"
  Bus Creator9/1 -> BMS_Modbus/1(BESS_MS), Memory/1
  [BESS_Inv_meas] -> Bus Creator9/2  "Inv_Meas_RTE"
  Bus Selector4/1 -> Bus Selector2/1  "<MN_CTRL>"
  Bus Selector4/2 -> Bus Selector6/1  "<IO_ctrl>"
  Bus Selector6/1 -> [Dout_GR3]  "<DOUT GR3>"
  Bus Selector2/2 -> [BESS_control]  "<Inv_Battery>"
  Bus Selector2/1 -> [enable]  "<Enable PWM>"
  Bus Selector2/5 -> [RTEvsSPS]  "<RTEvsSPS>"
  [remote_sense_RTE] -> Controller Mapping/4(HIL Outputs2)
  [Dout_GR3] -> Controller Mapping/5(Console Input)
  Controller Mapping/5(Gate Drive) -> [BESS_GateDrive]
  Controller Mapping/6(Gate Drive RTE) -> [BESSGateDriveRTE]
  [BESS_control] -> Bus Selector1/1
  [enable] -> Controller Mapping/1(En)
  Inverter_Batt_RTE/1(m) -> [BESS_Inv_meas]
  [BESS_Inv_meas] -> Controller Mapping/2(HIL Outputs)
  [BESS_GateDrive] -> Bus Selector12/1
  Bus Selector1/1 -> Switch1/1  "<Precharge>"
  Bus Selector1/2 -> Switch2/1  "<DC_Contactor>"
  Bus Selector1/3 -> Switch1/2, Switch2/2  "<Console_Ctrl>"
  Switch1/1 -> Contactors1/1(Precharge)
  Switch2/1 -> Contactors1/2(Main Contactor)
  Bus Selector2/3 -> Switch3/1  "<MX1>"
  [BESS_control] -> Bus Selector10/1
  Bus Selector10/1 -> Switch3/2, Switch4/2  "<Console_Ctrl>"
  Switch3/1 -> [BESS_MX1_ctrl]
  Controller Mapping/3(MX1 Main AC) -> Switch6/2, Switch6/1
  Switch4/1 -> [BESS_MX2_ctrl]
  Bus Selector2/4 -> Switch4/1  "<MX2>"
  Controller Mapping/4(MX2 Remote AC) -> Switch7/1, Switch7/2
  Bus Selector2/6 -> [LOCALvsREMOTE]  "<LOCALvsREMOTE>"
  [remote_sense_RTE] -> Switch5/1
  [BESS_local_sense] -> Switch5/3, Controller Mapping/6(HIL Outputs3)
  [LOCALvsREMOTE] -> Switch5/2
  Switch6/1 -> Switch3/3
  Constant/1 -> Switch6/3, Switch7/3
  Switch7/1 -> Switch4/3
  [BESS_MX1_meas] -> Bus Selector11/1
  Bus Selector11/1 -> Controller Mapping/7(HIL Outputs4)  "<Vabc_line>"
  Controller Mapping/1(Precharge) -> [BESS_precharge]
  [BESS_precharge] -> Switch1/3
  Controller Mapping/2(DC Contactor) -> [BESS_dc_contactor]
  [BESS_dc_contactor] -> Switch2/3
  Memory/1 -> monitoring/1
  Battery/1 -> [Battery]
  connections:
  LCL Filter 200kW1/RConn1 -- Inverter_Batt_RTE/LConn1
  LCL Filter 200kW1/RConn3 -- Inverter_Batt_RTE/LConn3
  LCL Filter 200kW1/RConn2 -- Inverter_Batt_RTE/LConn2
  Inverter_Batt_RTE/RConn1 -- Contactors1/LConn1
  Inverter_Batt_RTE/RConn2 -- Contactors1/LConn2
  1/0AWG_L1/RConn3 -- Breaker1/LConn3
  1/0AWG_L1/RConn2 -- Breaker1/LConn2
  1/0AWG_L1/RConn1 -- Breaker1/LConn1
  A/RConn1 -- 500kcmil-Mutual4/LConn1
  B/RConn1 -- 500kcmil-Mutual4/LConn2
  C/RConn1 -- 500kcmil-Mutual4/LConn3
  Breaker1/RConn2 -- SSN Interface Block (3ph)3/LConn2
  Breaker1/RConn3 -- SSN Interface Block (3ph)3/LConn3
  Breaker1/RConn1 -- SSN Interface Block (3ph)3/LConn1
  500kcmil-Mutual4/RConn1 -- 1/0AWG_L1/LConn1
  500kcmil-Mutual4/RConn2 -- 1/0AWG_L1/LConn2
  500kcmil-Mutual4/RConn3 -- 1/0AWG_L1/LConn3
  DC Voltage Source1/RConn1 -- Contactors1/RConn1
  DC Voltage Source1/LConn1 -- Contactors1/RConn2
  SSN Interface Block (3ph)3/RConn1 -- LCL Filter 200kW1/LConn1
  SSN Interface Block (3ph)3/RConn2 -- LCL Filter 200kW1/LConn2
  SSN Interface Block (3ph)3/RConn3 -- LCL Filter 200kW1/LConn3

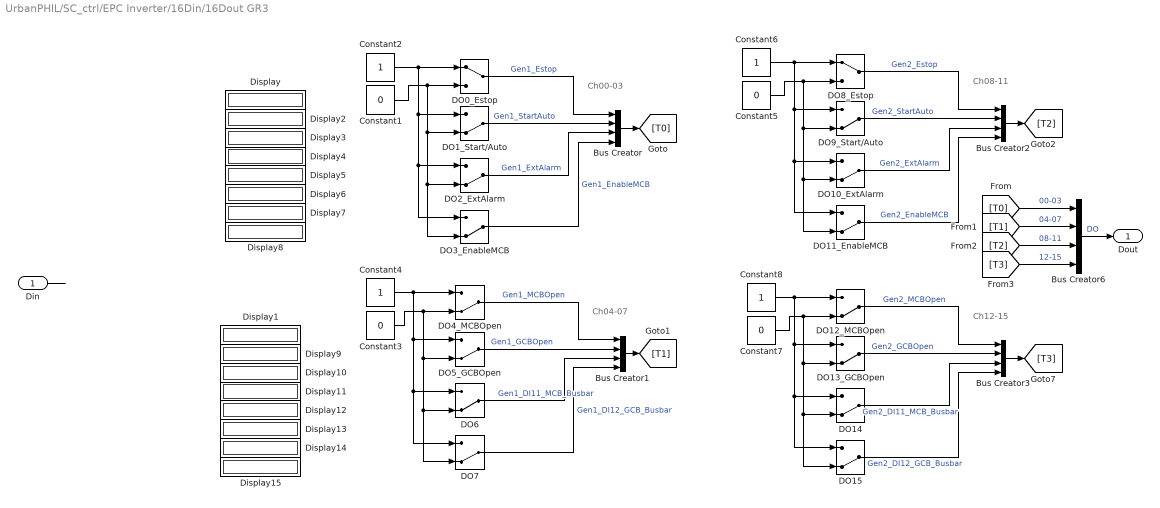
== system UrbanPHIL/SC_ctrl/EPC Inverter/16Din/16Dout GR3 ==
  note: Ch12-15
  note: Ch08-11
  note: Ch04-07
  note: Ch00-03
  Din : Inport
  Bus Creator{,1..3,6} (5 alike) : BusCreator
  Constant{1,3,5,7} (4 alike) : Constant  Value=0
  Constant{2,4,6,8} (4 alike) : Constant
  DO0_Estop : ManualSwitch
  DO10_ExtAlarm : ManualSwitch  CurrentSetting=0
  DO11_EnableMCB : ManualSwitch  CurrentSetting=0
  DO12_MCBOpen : ManualSwitch  CurrentSetting=0
  DO13_GCBOpen : ManualSwitch  CurrentSetting=0
  DO{6..7,14..15} (4 alike) : ManualSwitch  CurrentSetting=0
  DO1_Start/Auto : ManualSwitch  CurrentSetting=0
  DO2_ExtAlarm : ManualSwitch  CurrentSetting=0
  DO3_EnableMCB : ManualSwitch  CurrentSetting=0
  DO4_MCBOpen : ManualSwitch  CurrentSetting=0
  DO5_GCBOpen : ManualSwitch  CurrentSetting=0
  DO8_Estop : ManualSwitch
  DO9_Start/Auto : ManualSwitch  CurrentSetting=0
  Display{,1..15} (16 alike) : Display
  Dout : Outport
  wires:
  ? -> Display7/1  "<Gen1_Alarm_AB>"
  ? -> Display4/1  "<Gen1_Open_GCB>"
  ? -> Display15/1  "<Gen2_Alarm_CF>"
  ? -> Display14/1  "<Gen2_Alarm_AB>"
  ? -> Display13/1  "<Gen2_Open_MCB>"
  ? -> Display12/1  "<Gen2_Close_MCB>"
  ? -> Display11/1  "<Gen2_Open_GCB>"
  ? -> Display10/1  "<Gen2_Close_GCB>"
  ? -> Display9/1  "<Gen2_Fuel>"
  ? -> Display1/1  "<Gen2_Starter>"
  ? -> ?  "<DI_CH08-15>"
  ? -> Display8/1  "<Gen1_Alarm_CF>"
  ? -> Display6/1  "<Gen1_Open_MCB>"
  ? -> Display5/1  "<Gen1_Close_MCB>"
  ? -> Display3/1  "<Gen1_Close_GCB>"
  ? -> Display2/1  "<Gen1_Fuel>"
  ? -> Display/1  "<Gen1_Starter>"
  ? -> ?  "<DI_CH00-07>"
  Din/1 -> ?
  [T3] -> Bus Creator6/4  "12-15"
  [T2] -> Bus Creator6/3  "08-11"
  [T1] -> Bus Creator6/2  "04-07"
  [T0] -> Bus Creator6/1  "00-03"
  Bus Creator2/1 -> [T2]
  Bus Creator3/1 -> [T3]
  Bus Creator1/1 -> [T1]
  Bus Creator/1 -> [T0]
  DO15/1 -> Bus Creator3/4  "Gen2_DI12_GCB_Busbar"
  DO14/1 -> Bus Creator3/3  "Gen2_DI11_MCB_Busbar"
  DO13_GCBOpen/1 -> Bus Creator3/2  "Gen2_GCBOpen"
  DO12_MCBOpen/1 -> Bus Creator3/1  "Gen2_MCBOpen"
  Constant7/1 -> DO12_MCBOpen/2, DO13_GCBOpen/2, DO15/2, DO14/2
  Constant8/1 -> DO12_MCBOpen/1, DO13_GCBOpen/1, DO15/1, DO14/1
  DO11_EnableMCB/1 -> Bus Creator2/4  "Gen2_EnableMCB"
  DO10_ExtAlarm/1 -> Bus Creator2/3  "Gen2_ExtAlarm"
  DO9_Start/Auto/1 -> Bus Creator2/2  "Gen2_StartAuto"
  DO8_Estop/1 -> Bus Creator2/1  "Gen2_Estop"
  Constant5/1 -> DO10_ExtAlarm/2, DO11_EnableMCB/2, DO9_Start/Auto/2, DO8_Estop/2
  Constant6/1 -> DO10_ExtAlarm/1, DO11_EnableMCB/1, DO9_Start/Auto/1, DO8_Estop/1
  DO7/1 -> Bus Creator1/4  "Gen1_DI12_GCB_Busbar"
  DO6/1 -> Bus Creator1/3  "Gen1_DI11_MCB_Busbar"
  DO5_GCBOpen/1 -> Bus Creator1/2  "Gen1_GCBOpen"
  DO4_MCBOpen/1 -> Bus Creator1/1  "Gen1_MCBOpen"
  Constant3/1 -> DO4_MCBOpen/2, DO5_GCBOpen/2, DO7/2, DO6/2
  Constant4/1 -> DO4_MCBOpen/1, DO5_GCBOpen/1, DO7/1, DO6/1
  DO3_EnableMCB/1 -> Bus Creator/4  "Gen1_EnableMCB"
  DO2_ExtAlarm/1 -> Bus Creator/3  "Gen1_ExtAlarm"
  DO1_Start/Auto/1 -> Bus Creator/2  "Gen1_StartAuto"
  DO0_Estop/1 -> Bus Creator/1  "Gen1_Estop"
  Constant1/1 -> DO2_ExtAlarm/2, DO3_EnableMCB/2, DO1_Start/Auto/2, DO0_Estop/2
  Constant2/1 -> DO2_ExtAlarm/1, DO3_EnableMCB/1, DO1_Start/Auto/1, DO0_Estop/1
  Bus Creator6/1 -> Dout/1  "DO"

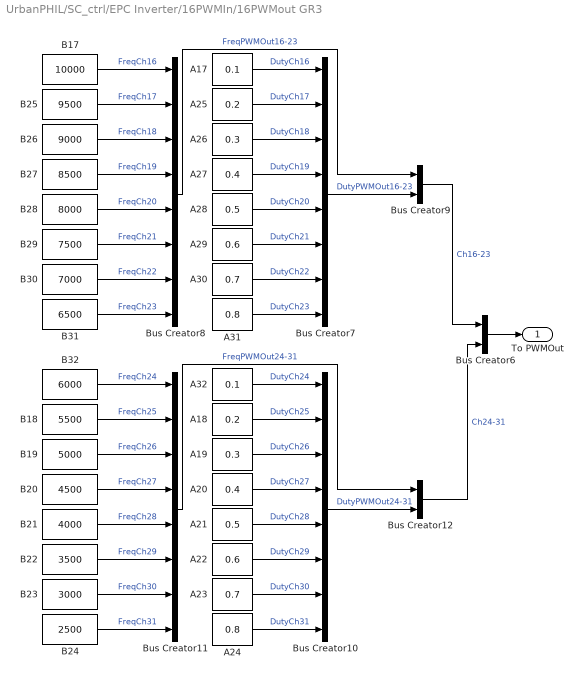
== system UrbanPHIL/SC_ctrl/EPC Inverter/16PWMIn/16PWMout GR3 ==
  A17 : Constant  Value=0.1
  A18 : Constant  Value=0.2
  A19 : Constant  Value=0.3
  A20 : Constant  Value=0.4
  A21 : Constant  Value=0.5
  A22 : Constant  Value=0.6
  A23 : Constant  Value=0.7
  A24 : Constant  Value=0.8
  A25 : Constant  Value=0.2
  A26 : Constant  Value=0.3
  A27 : Constant  Value=0.4
  A28 : Constant  Value=0.5
  A29 : Constant  Value=0.6
  A30 : Constant  Value=0.7
  A31 : Constant  Value=0.8
  A32 : Constant  Value=0.1
  B17 : Constant  Value=10000
  B18 : Constant  Value=5500
  B19 : Constant  Value=5000
  B20 : Constant  Value=4500
  B21 : Constant  Value=4000
  B22 : Constant  Value=3500
  B23 : Constant  Value=3000
  B24 : Constant  Value=2500
  B25 : Constant  Value=9500
  B26 : Constant  Value=9000
  B27 : Constant  Value=8500
  B28 : Constant  Value=8000
  B29 : Constant  Value=7500
  B30 : Constant  Value=7000
  B31 : Constant  Value=6500
  B32 : Constant  Value=6000
  Bus Creator{7..8,10..11} (4 alike) : BusCreator  Inputs=8
  Bus Creator12 : BusCreator  Inputs=2
  Bus Creator6 : BusCreator  Inputs=2
  Bus Creator9 : BusCreator  Inputs=2
  To PWMOut : Outport
  wires:
  Bus Creator9/1 -> Bus Creator6/1  "Ch16-23"
  Bus Creator12/1 -> Bus Creator6/2  "Ch24-31"
  Bus Creator11/1 -> Bus Creator12/1  "FreqPWMOut24-31"
  Bus Creator10/1 -> Bus Creator12/2  "DutyPWMOut24-31"
  B24/1 -> Bus Creator11/8  "FreqCh31"
  B23/1 -> Bus Creator11/7  "FreqCh30"
  B22/1 -> Bus Creator11/6  "FreqCh29"
  B21/1 -> Bus Creator11/5  "FreqCh28"
  B20/1 -> Bus Creator11/4  "FreqCh27"
  B19/1 -> Bus Creator11/3  "FreqCh26"
  B18/1 -> Bus Creator11/2  "FreqCh25"
  B32/1 -> Bus Creator11/1  "FreqCh24"
  A24/1 -> Bus Creator10/8  "DutyCh31"
  A23/1 -> Bus Creator10/7  "DutyCh30"
  A22/1 -> Bus Creator10/6  "DutyCh29"
  A21/1 -> Bus Creator10/5  "DutyCh28"
  A20/1 -> Bus Creator10/4  "DutyCh27"
  A19/1 -> Bus Creator10/3  "DutyCh26"
  A18/1 -> Bus Creator10/2  "DutyCh25"
  A32/1 -> Bus Creator10/1  "DutyCh24"
  Bus Creator8/1 -> Bus Creator9/1  "FreqPWMOut16-23"
  Bus Creator7/1 -> Bus Creator9/2  "DutyPWMOut16-23"
  B31/1 -> Bus Creator8/8  "FreqCh23"
  B30/1 -> Bus Creator8/7  "FreqCh22"
  B29/1 -> Bus Creator8/6  "FreqCh21"
  B28/1 -> Bus Creator8/5  "FreqCh20"
  B27/1 -> Bus Creator8/4  "FreqCh19"
  B26/1 -> Bus Creator8/3  "FreqCh18"
  B25/1 -> Bus Creator8/2  "FreqCh17"
  B17/1 -> Bus Creator8/1  "FreqCh16"
  A31/1 -> Bus Creator7/8  "DutyCh23"
  A30/1 -> Bus Creator7/7  "DutyCh22"
  A29/1 -> Bus Creator7/6  "DutyCh21"
  A28/1 -> Bus Creator7/5  "DutyCh20"
  A27/1 -> Bus Creator7/4  "DutyCh19"
  A26/1 -> Bus Creator7/3  "DutyCh18"
  A25/1 -> Bus Creator7/2  "DutyCh17"
  A17/1 -> Bus Creator7/1  "DutyCh16"
  Bus Creator6/1 -> To PWMOut/1

== system UrbanPHIL/SC_ctrl/EPC Inverter/16TSDIn/16 TSDOut GR3 ==
  Bus Creator1 : BusCreator  Inputs=3
  Din/Dout ch16-23 : Subsystem
  Din/Dout ch24-31 : Subsystem
  Dout state ctrl : Subsystem
  TSDout : Outport
  wires:
  Bus Creator1/1 -> TSDout/1
  Dout state ctrl/1(Event State OUT) -> Bus Creator1/3  "states"
  Din/Dout ch16-23/1(Out1) -> Bus Creator1/1  "times CH16-23"
  Din/Dout ch24-31/1(Out1) -> Bus Creator1/2  "times CH24-31"

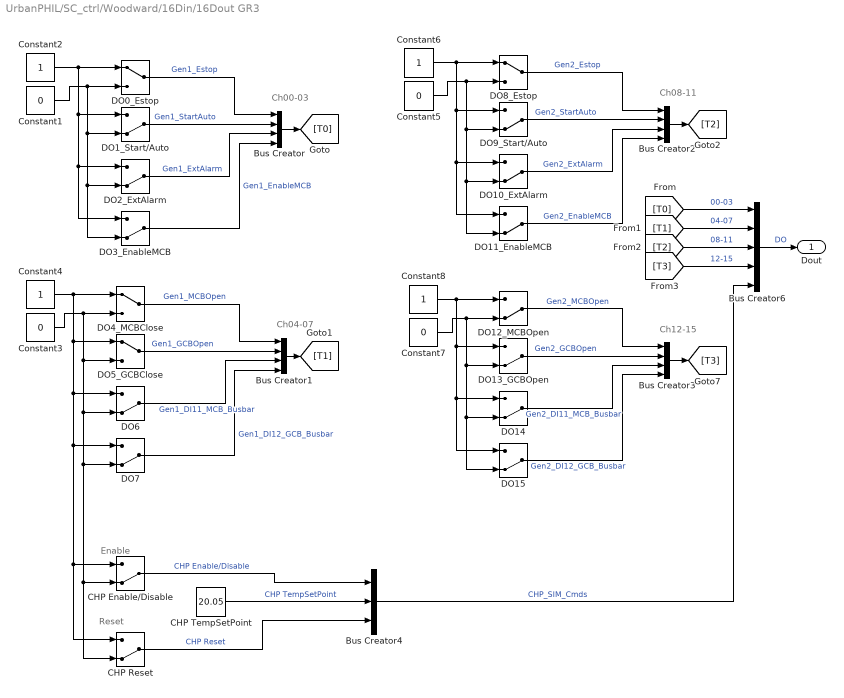
== system UrbanPHIL/SC_ctrl/Woodward/16Din/16Dout GR3 ==
  note: Ch00-03
  note: Ch04-07
  note: Ch08-11
  note: Ch12-15
  note: Enable
  note: Reset
  Bus Creator{,1..3} (4 alike) : BusCreator
  Bus Creator4 : BusCreator  Inputs=3
  Bus Creator6 : BusCreator  Inputs=5
  CHP Enable/Disable : ManualSwitch  CurrentSetting=0
  CHP Reset : ManualSwitch  CurrentSetting=0
  CHP TempSetPoint : Constant  Value=20.05
  Constant{1,3,5,7} (4 alike) : Constant  Value=0
  Constant{2,4,6,8} (4 alike) : Constant
  DO0_Estop : ManualSwitch
  DO10_ExtAlarm : ManualSwitch  CurrentSetting=0
  DO11_EnableMCB : ManualSwitch  CurrentSetting=0
  DO12_MCBOpen : ManualSwitch  CurrentSetting=0
  DO13_GCBOpen : ManualSwitch  CurrentSetting=0
  DO{6..7,14..15} (4 alike) : ManualSwitch  CurrentSetting=0
  DO1_Start/Auto : ManualSwitch  CurrentSetting=0
  DO2_ExtAlarm : ManualSwitch  CurrentSetting=0
  DO3_EnableMCB : ManualSwitch  CurrentSetting=0
  DO4_MCBClose : ManualSwitch
  DO5_GCBClose : ManualSwitch
  DO8_Estop : ManualSwitch
  DO9_Start/Auto : ManualSwitch  CurrentSetting=0
  Dout : Outport
  wires:
  Bus Creator4/1 -> Bus Creator6/5  "CHP_SIM_Cmds"
  CHP Reset/1 -> Bus Creator4/3  "CHP Reset"
  CHP TempSetPoint/1 -> Bus Creator4/2  "CHP TempSetPoint"
  CHP Enable/Disable/1 -> Bus Creator4/1  "CHP Enable/Disable"
  Bus Creator6/1 -> Dout/1  "DO"
  Constant2/1 -> DO0_Estop/1, DO1_Start/Auto/1, DO3_EnableMCB/1, DO2_ExtAlarm/1
  Constant1/1 -> DO0_Estop/2, DO1_Start/Auto/2, DO3_EnableMCB/2, DO2_ExtAlarm/2
  DO0_Estop/1 -> Bus Creator/1  "Gen1_Estop"
  DO1_Start/Auto/1 -> Bus Creator/2  "Gen1_StartAuto"
  DO2_ExtAlarm/1 -> Bus Creator/3  "Gen1_ExtAlarm"
  DO3_EnableMCB/1 -> Bus Creator/4  "Gen1_EnableMCB"
  Constant4/1 -> DO6/1, DO7/1, CHP Enable/Disable/1, CHP Reset/1, DO5_GCBClose/1, DO4_MCBClose/1
  Constant3/1 -> DO6/2, CHP Enable/Disable/2, CHP Reset/2, DO7/2, DO5_GCBClose/2, DO4_MCBClose/2
  DO4_MCBClose/1 -> Bus Creator1/1  "Gen1_MCBOpen"
  DO5_GCBClose/1 -> Bus Creator1/2  "Gen1_GCBOpen"
  DO6/1 -> Bus Creator1/3  "Gen1_DI11_MCB_Busbar"
  DO7/1 -> Bus Creator1/4  "Gen1_DI12_GCB_Busbar"
  Constant6/1 -> DO8_Estop/1, DO9_Start/Auto/1, DO11_EnableMCB/1, DO10_ExtAlarm/1
  Constant5/1 -> DO8_Estop/2, DO9_Start/Auto/2, DO11_EnableMCB/2, DO10_ExtAlarm/2
  DO8_Estop/1 -> Bus Creator2/1  "Gen2_Estop"
  DO9_Start/Auto/1 -> Bus Creator2/2  "Gen2_StartAuto"
  DO10_ExtAlarm/1 -> Bus Creator2/3  "Gen2_ExtAlarm"
  DO11_EnableMCB/1 -> Bus Creator2/4  "Gen2_EnableMCB"
  Constant8/1 -> DO14/1, DO15/1, DO13_GCBOpen/1, DO12_MCBOpen/1
  Constant7/1 -> DO14/2, DO15/2, DO13_GCBOpen/2, DO12_MCBOpen/2
  DO12_MCBOpen/1 -> Bus Creator3/1  "Gen2_MCBOpen"
  DO13_GCBOpen/1 -> Bus Creator3/2  "Gen2_GCBOpen"
  DO14/1 -> Bus Creator3/3  "Gen2_DI11_MCB_Busbar"
  DO15/1 -> Bus Creator3/4  "Gen2_DI12_GCB_Busbar"
  Bus Creator/1 -> [T0]
  Bus Creator1/1 -> [T1]
  Bus Creator3/1 -> [T3]
  Bus Creator2/1 -> [T2]
  [T0] -> Bus Creator6/1  "00-03"
  [T1] -> Bus Creator6/2  "04-07"
  [T2] -> Bus Creator6/3  "08-11"
  [T3] -> Bus Creator6/4  "12-15"

== system UrbanPHIL/SS_PV_BESS/EPC/BMS_Modbus ==
  BESS_MS : Inport
  Bus Selector : BusSelector  OutputSignals=Battery_Meas.SOC (%),Battery_Meas.Current (A),Battery_Meas.Voltage (V),BESS_MX1.cb_ms.Status,BESS_MX1.VRMSLL,BESS_MX1.Freq,BESS_MX1.kw,BESS_MX1.kvar
  Gain : Gain  Gain=100
  Gain1 : Gain  Gain=100
  Modbus device6 : rtio_generic_modbus/Modbus device  conf_name=EPC_BMS_cfg.opal  conf_name_mask=EPC_BMS_cfg.xls  sample_time=Ts
  Mux : Mux  Inputs=8
  wires:
  Bus Selector/7 -> Mux/7  "<kw>"
  Bus Selector/5 -> Mux/5  "<VRMSLL>"
  Bus Selector/1 -> Gain/1  "<SOC (%)>"
  Bus Selector/6 -> Gain1/1  "<Freq>"
  Bus Selector/8 -> Mux/8  "<kvar>"
  BESS_MS/1 -> Bus Selector/1
  Gain/1 -> Mux/1
  Bus Selector/3 -> Mux/3  "<Voltage (V)>"
  Bus Selector/2 -> Mux/2  "<Current (A)>"
  Bus Selector/4 -> Mux/4  "<Status>"
  Gain1/1 -> Mux/6
  Mux/1 -> Modbus device6/1

== system UrbanPHIL/SS_PV_BESS/EPC/Contactors1 ==
  note: with 10ohm resistor
  note: changed to 1000
      | to slow down the time
  Precharge : Inport
  Main Contactor : Inport  Port=2
  Brk_Battery : powerlib/Power Electronics/Ideal Switch  Ron=0.001  Lon=0  IC=0  Rs=1e6  Cs=inf  Measurements=on
  Brk_Precharge : powerlib/Power Electronics/Ideal Switch  Ron=1  Lon=0  IC=0  Rs=1e6  Cs=inf  Measurements=on
  DC+ Source : PMIOPort  Port=1  Side=Right
  DC+ Bus : PMIOPort  Port=2  Side=Left
  DC- Source : PMIOPort  Port=3  Side=Left
  DC- Bus : PMIOPort  Port=4  Side=Right
  wires:
  Precharge/1 -> Brk_Precharge/1
  Main Contactor/1 -> Brk_Battery/1
  connections:
  Brk_Battery/LConn1 -- DC+ Bus/RConn1 -- Brk_Precharge/LConn1
  Brk_Battery/RConn1 -- DC+ Source/RConn1 -- Brk_Precharge/RConn1
  DC- Bus/RConn1 -- DC- Source/RConn1
